simulink model "task6-Simulink"  (R2015b)
settings: Solver=ode23t  StartTime=0.0  StopTime=1  RelTol=1e-3
values from neighbouring files (symbols this model uses):
  A = [0 0 0 1 0 0;     0 0 0 0 1 0;      0 0 0 0 0 1;     (kt-ko)/J1 kt/(J1*n^2) -kt/J1 (dt-do)/J1 dt/(J1*n^2) -dt/J1;    -kt/(Jmg*n^2) -kt/((n^4)*Jmg) kt/((n^2)*Jmg) -dt/(Jmg*n^2) 1/Jmg*(-Km*Kemf/R-dt/(n^4)) dt/(n^2*Jmg);    kt/Jout kt/((n^2)*Jout) (-kt-kr)/Jout dt/Jout dt/((n^2)*Jout) -(dt+dj)/Jout]    [All Tasks Compiled.m]
  B = [0 0 0 0 Km/(R*Jmg) 0]'    [All Tasks Compiled.m]
  C = eye(6)    [All Tasks Compiled.m]
  D = [0 0 0 0 0 0]'    [All Tasks Compiled.m]
settings Model: Creator=atang  LastModifiedBy=daniella.a

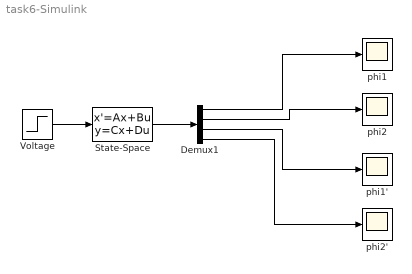
== system task6-Simulink ==
  Demux1 : Demux
  State-Space : StateSpace  A=A  B=B  C=C  D=D  X0=0
  Voltage : Step  Time=0  SampleTime=0
  phi1 : Scope
  phi1' : Scope
  phi2 : Scope
  phi2' : Scope
  wires:
  Voltage/1 -> State-Space/1
  State-Space/1 -> Demux1/1
  Demux1/1 -> phi1/1
  Demux1/2 -> phi2/1
  Demux1/3 -> phi1'/1
  Demux1/4 -> phi2'/1
